simulink model "mix_fl_01"  (Simulink 8.6)
settings: Solver=VariableStepAuto  StartTime=1  StopTime=1.7  MaxStep=0.000001  RelTol=1e-3
values from neighbouring files (symbols this model uses):
  delay_1 = r{1}./c    [mux_fl_01.m]
  delay_2 = r{2}./c    [mux_fl_01.m]
  delay_3 = r{3}./c    [mux_fl_01.m]
libraries: commsynccomp2 x49, simulink x49, dsparch4 x6, commchan3 x3
settings Model: Creator=my88899  LastModifiedBy=my88899
settings SolverCC: InitialStep=0.000001
settings DataIOCC: SaveFormat=Dataset  SignalLoggingSaveFormat=Dataset
settings OptimizationCC: ExpressionDepthLimit=128
settings DebuggingCC: UnderspecifiedInitializationDetection=Simplified  MergeDetectMultiDrivingBlocksExec=error  SolverPrmCheckMsg=none  FcnCallInpInsideContextMsg=EnableAllAsError  StateNameClashWarn=none
settings HardwareCC: ProdBitPerPointer=64  ProdLargestAtomicFloat=Float  ProdIntDivRoundTo=Zero  ProdEndianess=LittleEndian  ProdWordSize=64  ProdHWDeviceType=Intel->x86-64 (Windows64)
settings GRTTargetCC: GeneratePreprocessorConditionals=Use local settings  CombineOutputUpdateFcns=on  GRTInterface=off
settings ConfigComp: CovModelRefEnable=off
settings ConfigurationSet: Description=SimMechanics 2G

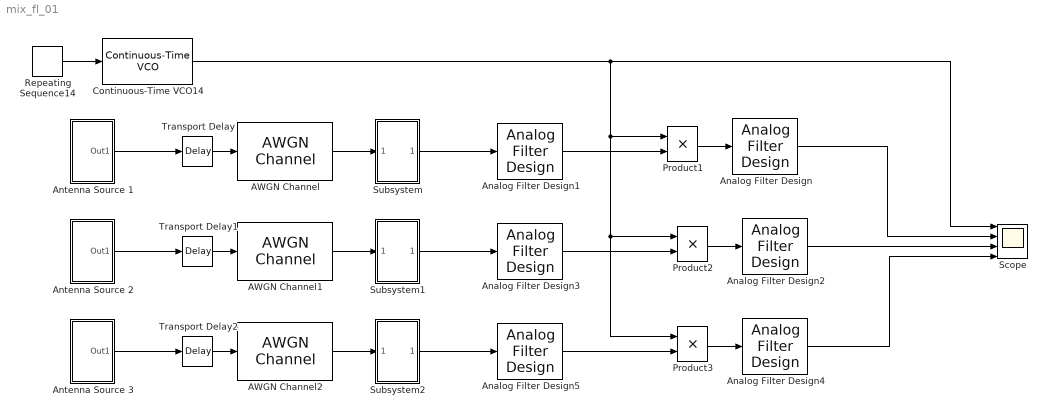
== system mix_fl_01 ==
  AWGN Channel : commchan3/AWGN Channel  InputProcessing=Columns as channels (frame based)  seed=67  noiseMode=Variance from mask  EbNodB=10  EsNodB=10  SNRdB=10  bitsPerSym=1  Ps=1  Tsym=1000000  variance=1
  AWGN Channel1 : commchan3/AWGN Channel  InputProcessing=Columns as channels (frame based)  seed=67  noiseMode=Variance from mask  EbNodB=10  EsNodB=10  SNRdB=10  bitsPerSym=1  Ps=1  Tsym=1000000  variance=1
  AWGN Channel2 : commchan3/AWGN Channel  InputProcessing=Columns as channels (frame based)  seed=67  noiseMode=Variance from mask  EbNodB=10  EsNodB=10  SNRdB=10  bitsPerSym=1  Ps=1  Tsym=1000000  variance=1
  Analog Filter Design : dsparch4/Analog Filter Design  method=Butterworth  filttype=Lowpass  N=12  Wlo=2*pi*20000  Whi=80  Rp=2  Rs=40
  Analog Filter Design1 : dsparch4/Analog Filter Design  method=Butterworth  filttype=Highpass  N=12  Wlo=2*pi*10000  Whi=80  Rp=2  Rs=40
  Analog Filter Design2 : dsparch4/Analog Filter Design  method=Butterworth  filttype=Lowpass  N=12  Wlo=2*pi*20000  Whi=80  Rp=2  Rs=40
  Analog Filter Design3 : dsparch4/Analog Filter Design  method=Butterworth  filttype=Highpass  N=12  Wlo=2*pi*10000  Whi=80  Rp=2  Rs=40
  Analog Filter Design4 : dsparch4/Analog Filter Design  method=Butterworth  filttype=Lowpass  N=12  Wlo=2*pi*20000  Whi=80  Rp=2  Rs=40
  Analog Filter Design5 : dsparch4/Analog Filter Design  method=Butterworth  filttype=Highpass  N=12  Wlo=2*pi*10000  Whi=80  Rp=2  Rs=40
  Antenna Source 1 : Subsystem
  Antenna Source 2 : Subsystem
  Antenna Source 3 : Subsystem
  Continuous-Time VCO14 : commsynccomp2/Continuous-Time VCO  Ac=5  Fc=100000  Kc=10000  Ph=0
  Product1 : Product
  Product2 : Product
  Product3 : Product
  Repeating Sequence14 : simulink/Sources/Repeating Sequence  rep_seq_t=[0 1]  rep_seq_y=[0 10]
  Scope : Scope  NumInputPorts=4
  Subsystem : Subsystem
  Subsystem1 : Subsystem
  Subsystem2 : Subsystem
  Transport Delay : TransportDelay  DelayTime=delay_1  BufferSize=3000000
  Transport Delay1 : TransportDelay  DelayTime=delay_2  BufferSize=3000000
  Transport Delay2 : TransportDelay  DelayTime=delay_3  BufferSize=3000000
  wires:
  Repeating Sequence14/1 -> Continuous-Time VCO14/1
  Product1/1 -> Analog Filter Design/1
  Transport Delay/1 -> AWGN Channel/1
  Analog Filter Design1/1 -> Product1/2
  AWGN Channel/1 -> Subsystem/1(In1)
  Transport Delay1/1 -> AWGN Channel1/1
  Transport Delay2/1 -> AWGN Channel2/1
  Analog Filter Design2/1 -> Scope/3
  Product2/1 -> Analog Filter Design2/1
  Analog Filter Design3/1 -> Product2/2
  AWGN Channel1/1 -> Subsystem1/1(In1)
  Continuous-Time VCO14/1 -> Product3/1, Product2/1, Product1/1, Scope/1
  Antenna Source 3/1(Out1) -> Transport Delay2/1
  Antenna Source 2/1(Out1) -> Transport Delay1/1
  Antenna Source 1/1(Out1) -> Transport Delay/1
  Analog Filter Design4/1 -> Scope/4
  Product3/1 -> Analog Filter Design4/1
  Analog Filter Design5/1 -> Product3/2
  AWGN Channel2/1 -> Subsystem2/1(In1)
  Subsystem/1(Out1) -> Analog Filter Design1/1
  Subsystem1/1(Out1) -> Analog Filter Design3/1
  Subsystem2/1(Out1) -> Analog Filter Design5/1
  Analog Filter Design/1 -> Scope/2

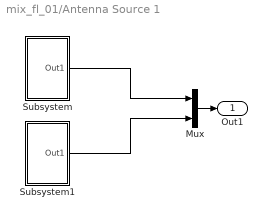
== system mix_fl_01/Antenna Source 1 ==
  Mux : Mux  Inputs=2
  Subsystem : Subsystem
  Subsystem1 : Subsystem
  Out1 : Outport
  wires:
  Mux/1 -> Out1/1
  Subsystem1/1(Out1) -> Mux/2
  Subsystem/1(Out1) -> Mux/1

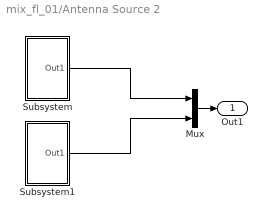
== system mix_fl_01/Antenna Source 2 ==
  Mux : Mux  Inputs=2
  Subsystem : Subsystem
  Subsystem1 : Subsystem
  Out1 : Outport
  wires:
  Subsystem/1(Out1) -> Mux/1
  Subsystem1/1(Out1) -> Mux/2
  Mux/1 -> Out1/1

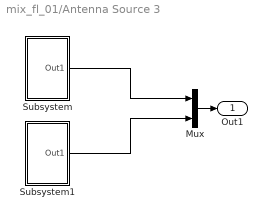
== system mix_fl_01/Antenna Source 3 ==
  Mux : Mux  Inputs=2
  Subsystem : Subsystem
  Subsystem1 : Subsystem
  Out1 : Outport
  wires:
  Subsystem/1(Out1) -> Mux/1
  Subsystem1/1(Out1) -> Mux/2
  Mux/1 -> Out1/1

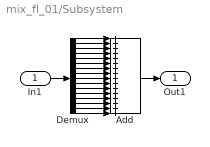
== system mix_fl_01/Subsystem ==
  In1 : Inport
  Add : Sum  Inputs=++++++++++++++++
  Demux : Demux  Outputs=16
  Out1 : Outport
  wires:
  Demux/6 -> Add/6
  Demux/7 -> Add/7
  Demux/3 -> Add/3
  Demux/9 -> Add/9
  Demux/2 -> Add/2
  Demux/5 -> Add/5
  Demux/8 -> Add/8
  Demux/4 -> Add/4
  Demux/10 -> Add/10
  Demux/1 -> Add/1
  Demux/12 -> Add/12
  Demux/15 -> Add/15
  Demux/13 -> Add/13
  Demux/14 -> Add/14
  Demux/16 -> Add/16
  Add/1 -> Out1/1
  In1/1 -> Demux/1
  Demux/11 -> Add/11

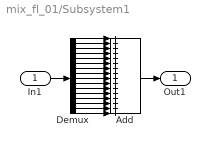
== system mix_fl_01/Subsystem1 ==
  In1 : Inport
  Add : Sum  Inputs=++++++++++++++++
  Demux : Demux  Outputs=16
  Out1 : Outport
  wires:
  Demux/11 -> Add/11
  In1/1 -> Demux/1
  Add/1 -> Out1/1
  Demux/16 -> Add/16
  Demux/14 -> Add/14
  Demux/13 -> Add/13
  Demux/15 -> Add/15
  Demux/12 -> Add/12
  Demux/1 -> Add/1
  Demux/10 -> Add/10
  Demux/4 -> Add/4
  Demux/8 -> Add/8
  Demux/5 -> Add/5
  Demux/2 -> Add/2
  Demux/9 -> Add/9
  Demux/3 -> Add/3
  Demux/7 -> Add/7
  Demux/6 -> Add/6

== system mix_fl_01/Subsystem2 ==
  In1 : Inport
  Add : Sum  Inputs=++++++++++++++++
  Demux : Demux  Outputs=16
  Out1 : Outport
  wires:
  Demux/6 -> Add/6
  Demux/7 -> Add/7
  Demux/3 -> Add/3
  Demux/9 -> Add/9
  Demux/2 -> Add/2
  Demux/5 -> Add/5
  Demux/8 -> Add/8
  Demux/4 -> Add/4
  Demux/10 -> Add/10
  Demux/1 -> Add/1
  Demux/12 -> Add/12
  Demux/15 -> Add/15
  Demux/13 -> Add/13
  Demux/14 -> Add/14
  Demux/16 -> Add/16
  Add/1 -> Out1/1
  In1/1 -> Demux/1
  Demux/11 -> Add/11

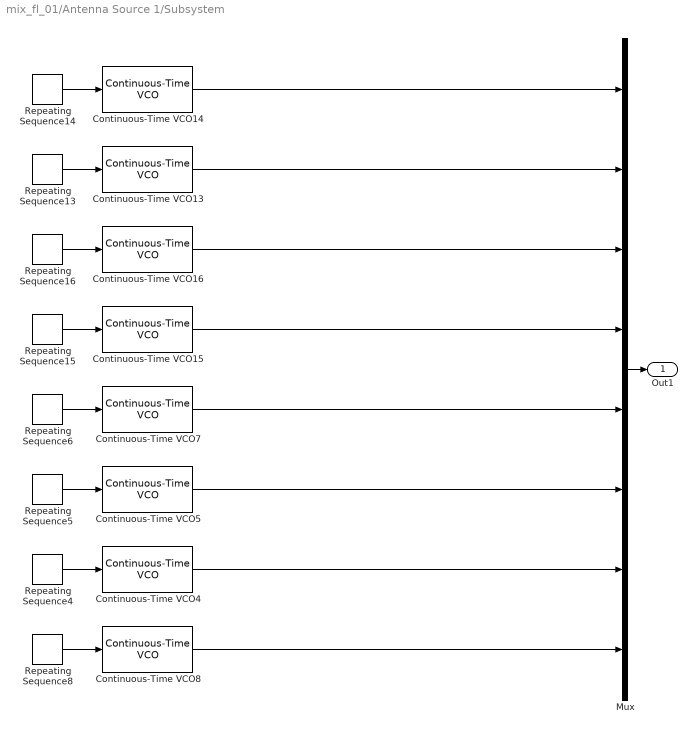
== system mix_fl_01/Antenna Source 1/Subsystem ==
  Continuous-Time VCO{4..5,7..8,13..16} (8 alike) : commsynccomp2/Continuous-Time VCO  Ac=5  Fc=100000  Kc=10000  Ph=0
  Mux : Mux  Inputs=8
  Repeating Sequence{4..6,8,13..16} (8 alike) : simulink/Sources/Repeating Sequence  rep_seq_t=[0 1]  rep_seq_y=[0 10]
  Out1 : Outport
  wires:
  Repeating Sequence5/1 -> Continuous-Time VCO5/1
  Continuous-Time VCO16/1 -> Mux/3
  Repeating Sequence8/1 -> Continuous-Time VCO8/1
  Repeating Sequence4/1 -> Continuous-Time VCO4/1
  Repeating Sequence6/1 -> Continuous-Time VCO7/1
  Continuous-Time VCO5/1 -> Mux/6
  Continuous-Time VCO13/1 -> Mux/2
  Continuous-Time VCO8/1 -> Mux/8
  Continuous-Time VCO7/1 -> Mux/5
  Continuous-Time VCO4/1 -> Mux/7
  Continuous-Time VCO15/1 -> Mux/4
  Mux/1 -> Out1/1
  Repeating Sequence13/1 -> Continuous-Time VCO13/1
  Repeating Sequence14/1 -> Continuous-Time VCO14/1
  Repeating Sequence15/1 -> Continuous-Time VCO15/1
  Repeating Sequence16/1 -> Continuous-Time VCO16/1
  Continuous-Time VCO14/1 -> Mux/1

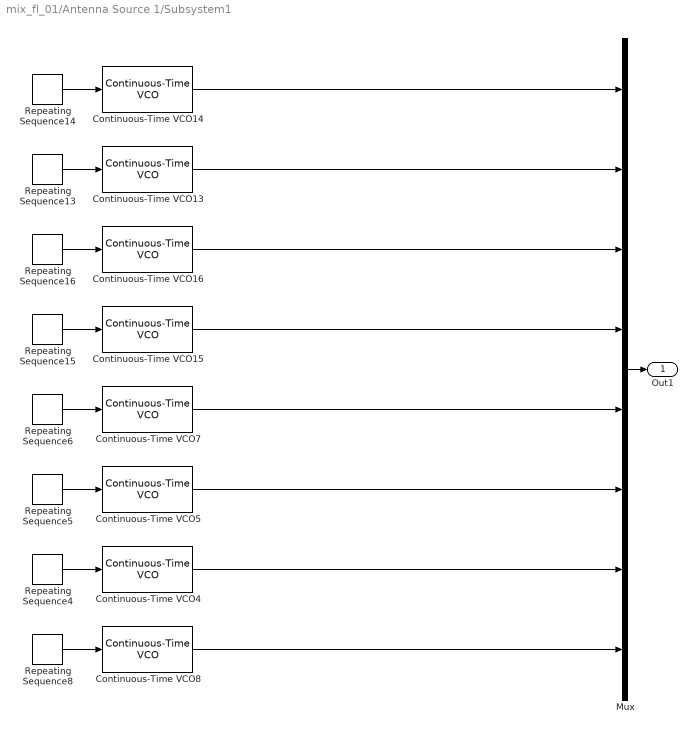
== system mix_fl_01/Antenna Source 1/Subsystem1 ==
  Continuous-Time VCO{4..5,7..8,13..16} (8 alike) : commsynccomp2/Continuous-Time VCO  Ac=5  Fc=100000  Kc=10000  Ph=0
  Mux : Mux  Inputs=8
  Repeating Sequence{4..6,8,13..16} (8 alike) : simulink/Sources/Repeating Sequence  rep_seq_t=[0 1]  rep_seq_y=[0 10]
  Out1 : Outport
  wires:
  Continuous-Time VCO14/1 -> Mux/1
  Repeating Sequence16/1 -> Continuous-Time VCO16/1
  Repeating Sequence15/1 -> Continuous-Time VCO15/1
  Repeating Sequence14/1 -> Continuous-Time VCO14/1
  Repeating Sequence13/1 -> Continuous-Time VCO13/1
  Mux/1 -> Out1/1
  Continuous-Time VCO15/1 -> Mux/4
  Continuous-Time VCO4/1 -> Mux/7
  Continuous-Time VCO7/1 -> Mux/5
  Continuous-Time VCO8/1 -> Mux/8
  Continuous-Time VCO13/1 -> Mux/2
  Continuous-Time VCO5/1 -> Mux/6
  Repeating Sequence6/1 -> Continuous-Time VCO7/1
  Repeating Sequence4/1 -> Continuous-Time VCO4/1
  Repeating Sequence8/1 -> Continuous-Time VCO8/1
  Continuous-Time VCO16/1 -> Mux/3
  Repeating Sequence5/1 -> Continuous-Time VCO5/1

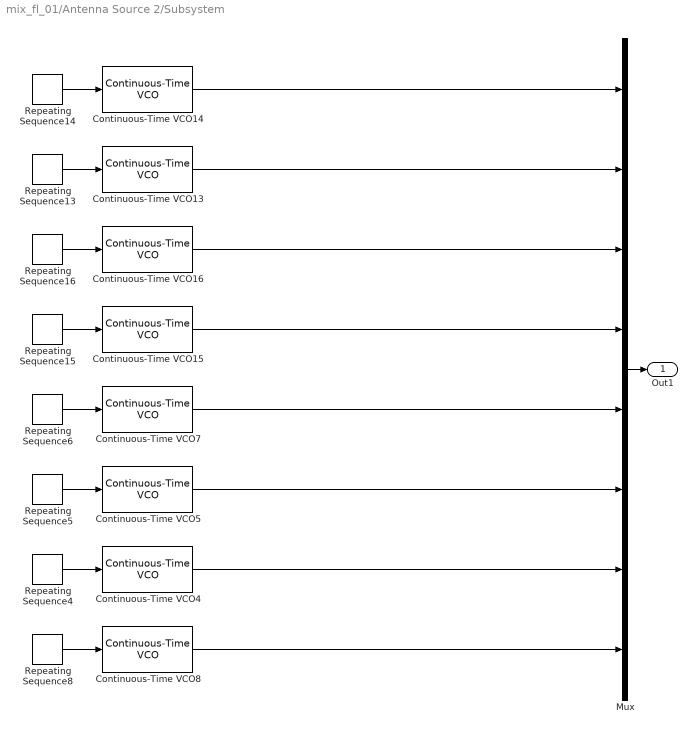
== system mix_fl_01/Antenna Source 2/Subsystem ==
  Continuous-Time VCO{4..5,7..8,13..16} (8 alike) : commsynccomp2/Continuous-Time VCO  Ac=5  Fc=100000  Kc=10000  Ph=0
  Mux : Mux  Inputs=8
  Repeating Sequence{4..6,8,13..16} (8 alike) : simulink/Sources/Repeating Sequence  rep_seq_t=[0 1]  rep_seq_y=[0 10]
  Out1 : Outport
  wires:
  Continuous-Time VCO14/1 -> Mux/1
  Repeating Sequence16/1 -> Continuous-Time VCO16/1
  Repeating Sequence15/1 -> Continuous-Time VCO15/1
  Repeating Sequence14/1 -> Continuous-Time VCO14/1
  Repeating Sequence13/1 -> Continuous-Time VCO13/1
  Mux/1 -> Out1/1
  Continuous-Time VCO15/1 -> Mux/4
  Continuous-Time VCO4/1 -> Mux/7
  Continuous-Time VCO7/1 -> Mux/5
  Continuous-Time VCO8/1 -> Mux/8
  Continuous-Time VCO13/1 -> Mux/2
  Continuous-Time VCO5/1 -> Mux/6
  Repeating Sequence6/1 -> Continuous-Time VCO7/1
  Repeating Sequence4/1 -> Continuous-Time VCO4/1
  Repeating Sequence8/1 -> Continuous-Time VCO8/1
  Continuous-Time VCO16/1 -> Mux/3
  Repeating Sequence5/1 -> Continuous-Time VCO5/1

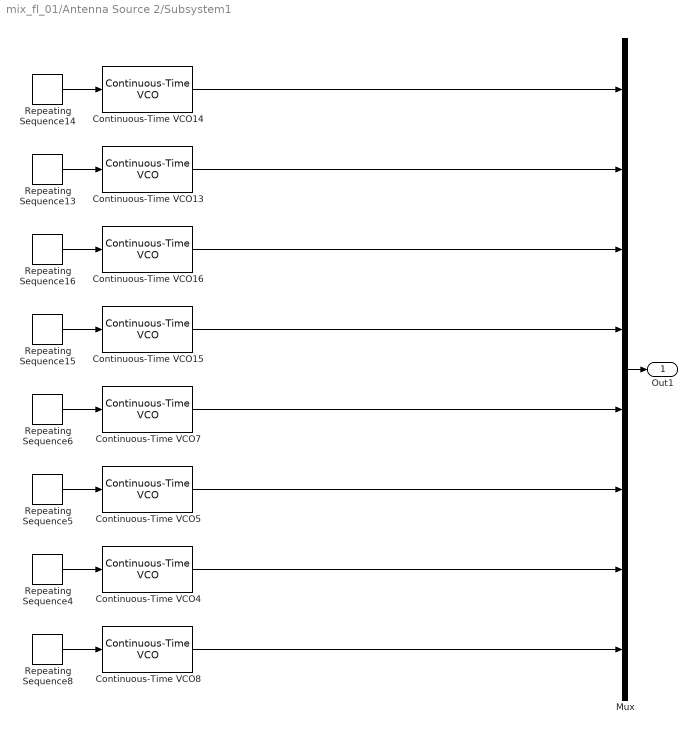
== system mix_fl_01/Antenna Source 2/Subsystem1 ==
  Continuous-Time VCO{4..5,7..8,13..16} (8 alike) : commsynccomp2/Continuous-Time VCO  Ac=5  Fc=100000  Kc=10000  Ph=0
  Mux : Mux  Inputs=8
  Repeating Sequence{4..6,8,13..16} (8 alike) : simulink/Sources/Repeating Sequence  rep_seq_t=[0 1]  rep_seq_y=[0 10]
  Out1 : Outport
  wires:
  Repeating Sequence5/1 -> Continuous-Time VCO5/1
  Continuous-Time VCO16/1 -> Mux/3
  Repeating Sequence8/1 -> Continuous-Time VCO8/1
  Repeating Sequence4/1 -> Continuous-Time VCO4/1
  Repeating Sequence6/1 -> Continuous-Time VCO7/1
  Continuous-Time VCO5/1 -> Mux/6
  Continuous-Time VCO13/1 -> Mux/2
  Continuous-Time VCO8/1 -> Mux/8
  Continuous-Time VCO7/1 -> Mux/5
  Continuous-Time VCO4/1 -> Mux/7
  Continuous-Time VCO15/1 -> Mux/4
  Mux/1 -> Out1/1
  Repeating Sequence13/1 -> Continuous-Time VCO13/1
  Repeating Sequence14/1 -> Continuous-Time VCO14/1
  Repeating Sequence15/1 -> Continuous-Time VCO15/1
  Repeating Sequence16/1 -> Continuous-Time VCO16/1
  Continuous-Time VCO14/1 -> Mux/1

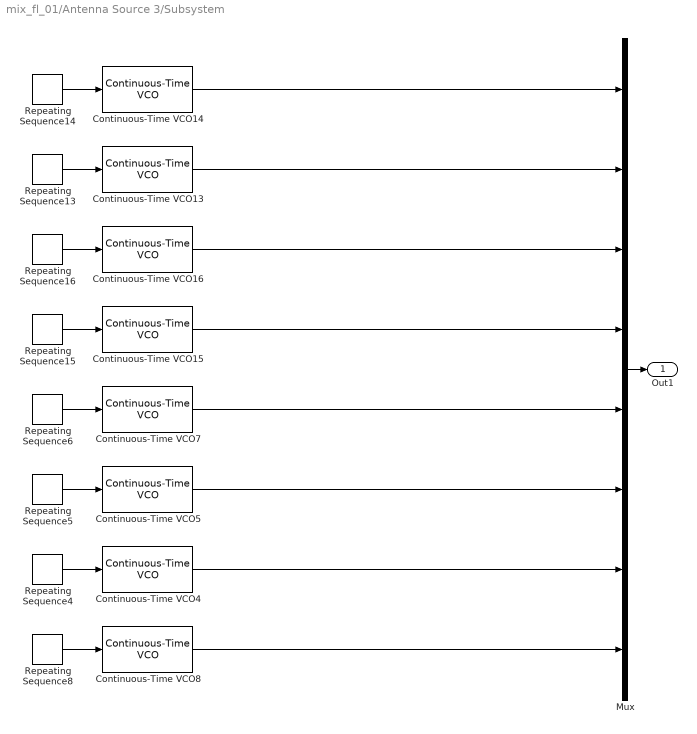
== system mix_fl_01/Antenna Source 3/Subsystem ==
  Continuous-Time VCO{4..5,7..8,13..16} (8 alike) : commsynccomp2/Continuous-Time VCO  Ac=5  Fc=100000  Kc=10000  Ph=0
  Mux : Mux  Inputs=8
  Repeating Sequence{4..6,8,13..16} (8 alike) : simulink/Sources/Repeating Sequence  rep_seq_t=[0 1]  rep_seq_y=[0 10]
  Out1 : Outport
  wires:
  Continuous-Time VCO14/1 -> Mux/1
  Repeating Sequence16/1 -> Continuous-Time VCO16/1
  Repeating Sequence15/1 -> Continuous-Time VCO15/1
  Repeating Sequence14/1 -> Continuous-Time VCO14/1
  Repeating Sequence13/1 -> Continuous-Time VCO13/1
  Mux/1 -> Out1/1
  Continuous-Time VCO15/1 -> Mux/4
  Continuous-Time VCO4/1 -> Mux/7
  Continuous-Time VCO7/1 -> Mux/5
  Continuous-Time VCO8/1 -> Mux/8
  Continuous-Time VCO13/1 -> Mux/2
  Continuous-Time VCO5/1 -> Mux/6
  Repeating Sequence6/1 -> Continuous-Time VCO7/1
  Repeating Sequence4/1 -> Continuous-Time VCO4/1
  Repeating Sequence8/1 -> Continuous-Time VCO8/1
  Continuous-Time VCO16/1 -> Mux/3
  Repeating Sequence5/1 -> Continuous-Time VCO5/1

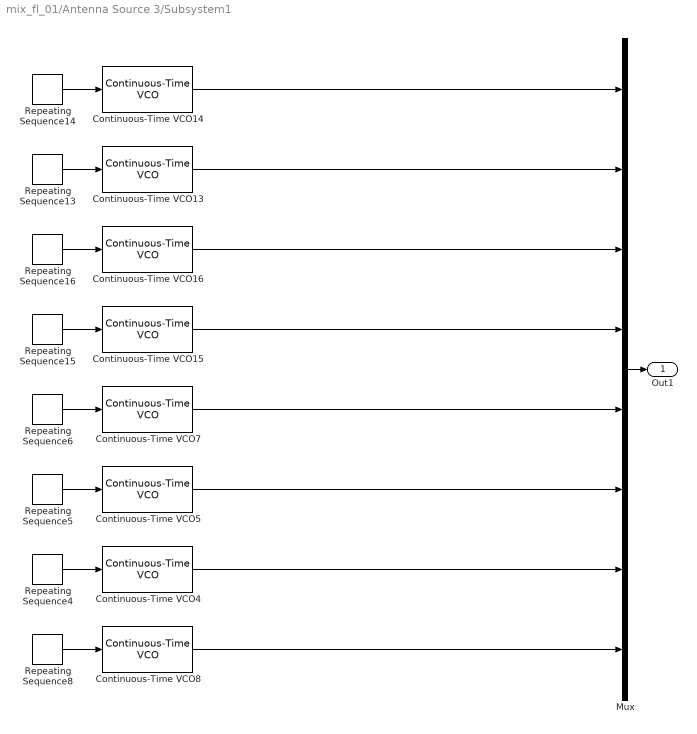
== system mix_fl_01/Antenna Source 3/Subsystem1 ==
  Continuous-Time VCO{4..5,7..8,13..16} (8 alike) : commsynccomp2/Continuous-Time VCO  Ac=5  Fc=100000  Kc=10000  Ph=0
  Mux : Mux  Inputs=8
  Repeating Sequence{4..6,8,13..16} (8 alike) : simulink/Sources/Repeating Sequence  rep_seq_t=[0 1]  rep_seq_y=[0 10]
  Out1 : Outport
  wires:
  Repeating Sequence5/1 -> Continuous-Time VCO5/1
  Continuous-Time VCO16/1 -> Mux/3
  Repeating Sequence8/1 -> Continuous-Time VCO8/1
  Repeating Sequence4/1 -> Continuous-Time VCO4/1
  Repeating Sequence6/1 -> Continuous-Time VCO7/1
  Continuous-Time VCO5/1 -> Mux/6
  Continuous-Time VCO13/1 -> Mux/2
  Continuous-Time VCO8/1 -> Mux/8
  Continuous-Time VCO7/1 -> Mux/5
  Continuous-Time VCO4/1 -> Mux/7
  Continuous-Time VCO15/1 -> Mux/4
  Mux/1 -> Out1/1
  Repeating Sequence13/1 -> Continuous-Time VCO13/1
  Repeating Sequence14/1 -> Continuous-Time VCO14/1
  Repeating Sequence15/1 -> Continuous-Time VCO15/1
  Repeating Sequence16/1 -> Continuous-Time VCO16/1
  Continuous-Time VCO14/1 -> Mux/1
